simulink model "dqn_C_PQ_HVsMC"  (R2024a)
settings: Solver=FixedStepDiscrete  StartTime=0.0  StopTime=10  FixedStep=Ts_Power  RelTol=1e-3
PreLoadFcn:
  | % HVDCMMCInterconnectionParam
StartFcn:
  | tic
StopFcn:
  | toc
values from neighbouring files (symbols this model uses):
  C_PM = 1.758e-3    (= 0.001758)    [dqnMMCsingle.m]
  Fnom = 50    [dqnMMCsingle.m]
  HRM = 1    [dqnMMCsingle.m]
  Ki_Ireg = 6    [dqnMMCsingle.m]
  Ki_Qreg = 1.0    (= 1)    [dqnMMCsingle.m]
  Kp_Ireg = 0.6    [dqnMMCsingle.m]
  Kp_Qreg = 0.5/3    (= 0.166666666667)    [dqnMMCsingle.m]
  Larm = Larm_pu*(Zb_ac/(2*pi*Fnom))    [dqnMMCsingle.m]
  Larm_pu = 0.15    [dqnMMCsingle.m]
  Lff = Larm_pu/2    (= 0.075)    [dqnMMCsingle.m]
  Limits_Ireg = [ 2.0  -2.0]    [dqnMMCsingle.m]
  Limits_Qreg = [ 0.25, -0.25 ]    [dqnMMCsingle.m]
  Limits_VDCreg = [ 2.0  -2.0]    [dqnMMCsingle.m]
  Lxfo = 0.12    [dqnMMCsingle.m]
  N = 1    [dqnMMCsingle.m]
  Nb_PM = 36    [dqnMMCsingle.m]
  Pnom = 1000e6    (= 1000000000)    [dqnMMCsingle.m]
  R_startup = 400    [dqnMMCsingle.m]
  Rarm = Rarm_pu*Zb_ac    [dqnMMCsingle.m]
  Rff = Rarm_pu/2    (= 0.00075)    [dqnMMCsingle.m]
  Rxfo = 0.003    [dqnMMCsingle.m]
  Slope_Qref = 0.5    [dqnMMCsingle.m]
  Slope_Vdc_ref = Vnom_dc/5    (= 128000)    [dqnMMCsingle.m]
  Tfault = 9999    [dqnMMCsingle.m]
  Ts = Ts_Control    (= 4e-05)    [dqnMMCsingle.m]
  Ts_Control = 40e-6    (= 4e-05)    [dqnMMCsingle.m]
  Ts_dqn = 2e-5    (= 2e-05)    [dqnMMCsingle.m]
  Ts_Power = 20e-6    (= 2e-05)    [dqnMMCsingle.m]
  Vnom_dc = 640e3    (= 640000)    [dqnMMCsingle.m]
  Vnom_prim = 400e3    (= 400000)    [dqnMMCsingle.m]
  Vnom_sec = 333e3    (= 333000)    [dqnMMCsingle.m]
  Ws = 2*pi*50    (= 314.159265359)    [dqnMMCsingle.m]
undefined symbols (not defined in the file or in its folder): DiscIntNeverNeededParam, Discrete, DQN_Lib, gcbh, Int_DQNc_Mat, Mult_DQNc_Mat, Pcc, S, sps, sps_rtmsupport, spsMeanValueVariableFrequencyModel, spsPLL3phModel, SY3
libraries: simulink x18, spsControlledVoltageSourceLib x15, spsVoltageMeasurementLib x9, powerlib_extras x6, spsSecondOrderFilterLib x6, spsCurrentMeasurementLib x6, spsIdealSwitchLib x6, spsMeanLib x4, spsdq0toabcLib x4, spsMeanVariableFrequencyLib x4, spsabctodq0Lib x4, spsThreePhaseSeriesRLCBranchLib x4
(part 6 of 6)

== matlab function dqn_C_PQ_HVsMC/DQsym/Mult_DQNc_Mat3 ==
  data: Xdcpnz_c input; Ydcpnz_c input; N parameter; HrmDbl parameter; Zdcpnz_c output
function Zdcpnz_c    = fMultDQNc(Xdcpnz_c, Ydcpnz_c, N, HrmDbl)
    Zdcpnz_c = complex(zeros(3,2*N+1));

    persistent T132;
    persistent T213;
    persistent T231;
    persistent T321;
    persistent T312;
    persistent Sas;
    persistent Ssa;

    if(isempty(T132)) 
        T132 = [1 0 0; 0 0 1; 0 1 0];
        T213 = [0 1 0; 1 0 0; 0 0 1];
        T231 = [0 1 0; 0 0 1; 1 0 0];
        T321 = [0 0 1; 0 1 0; 1 0 0];
        T312 = [0 0 1; 1 0 0; 0 1 0];

        a = -0.5+0.866i;
        a2 = -0.5-0.866i;
        Sas = [1,a,a2;1,a2,a;1,1,1]/3;
        Ssa = eye(3)/(Sas);
    end

%%%%%%%%%%%%%%%%%%%%%%%%%%%%%%

    Zdcpnz_c(:,1) = Sas*(Ssa*Xdcpnz_c(:,1).*Ssa*Ydcpnz_c(:,1));

    sX = size(Xdcpnz_c,2);
    Xdcpnz_c = [Xdcpnz_c zeros(3,N+1-sX)];

    sY = size(Ydcpnz_c,2);
    Ydcpnz_c = [Ydcpnz_c zeros(3,N+1-sY)];

       
    for h = 1 : 2*N
        if(h<=N)

            Zdcpnz_c(3,1) = Zdcpnz_c(3,1) + 0.5*real(Xdcpnz_c(:,h+1)'*Ydcpnz_c(:,h+1));


            Zdcpnz_c(3,2*h+1) = Zdcpnz_c(3,2*h+1) + 0.5*Xdcpnz_c(1,h+1)*Ydcpnz_c(2,h+1)*exp(-1i*pi/2);

            Zdcpnz_c(1:2,1) = Zdcpnz_c(1:2,1) + 0.25*abs(Xdcpnz_c(1,h+1))*abs(Ydcpnz_c(2,h+1))*[1;1].*exp(1i*((-angle(Xdcpnz_c(1,h+1))+angle(Ydcpnz_c(2,h+1)))*[1;-1]));
            Zdcpnz_c(1:2,1) = Zdcpnz_c(1:2,1) + 0.25*abs(Xdcpnz_c(1,h+1))*abs(Ydcpnz_c(3,h+1))*[1;1].*exp(1i*((-angle(Xdcpnz_c(1,h+1))+angle(Ydcpnz_c(3,h+1)))*[-1;1]));


            Zdcpnz_c(3,2*h+1) = Zdcpnz_c(3,2*h+1) + 0.5*Xdcpnz_c(2,h+1)*Ydcpnz_c(1,h+1)*exp(-1i*pi/2);


            Zdcpnz_c(1:2,1) = Zdcpnz_c(1:2,1) + 0.25*abs(Xdcpnz_c(2,h+1))*abs(Ydcpnz_c(1,h+1))*[1;1].*exp(1i*((-angle(Xdcpnz_c(2,h+1))+angle(Ydcpnz_c(1,h+1)))*[-1;1]));
            Zdcpnz_c(1:2,1) = Zdcpnz_c(1:2,1) + 0.25*abs(Xdcpnz_c(2,h+1))*abs(Ydcpnz_c(3,h+1))*[1;1].*exp(1i*((-angle(Xdcpnz_c(2,h+1))+angle(Ydcpnz_c(3,h+1)))*[1;-1]));
            
            Zdcpnz_c(1:2,1) = Zdcpnz_c(1:2,1) + 0.25*abs(Xdcpnz_c(3,h+1))*abs(Ydcpnz_c(1,h+1))*[1;1].*exp(1i*((-angle(Xdcpnz_c(3,h+1))+angle(Ydcpnz_c(1,h+1)))*[1;-1]));
            Zdcpnz_c(1:2,1) = Zdcpnz_c(1:2,1) + 0.25*abs(Xdcpnz_c(3,h+1))*abs(Ydcpnz_c(2,h+1))*[1;1].*exp(1i*((-angle(Xdcpnz_c(3,h+1))+angle(Ydcpnz_c(2,h+1)))*[-1;+1]));

            %%%%%%%%%%%%%%%%% POSITIVE (Ydc*Xp) %%%%%%%%%%%%%%%%%%%
            Zdcpnz_c(:,h+1) = Zdcpnz_c(:,h+1) + T312*Ydcpnz_c(:,1)*Xdcpnz_c(1,h+1); %[0 0 1; 1 0 0; 0 1 0]
            %%%%%%%%%%%%%%%%% POSITIVE (Xdc*Yp) %%%%%%%%%%%%%%%%%%%
            Zdcpnz_c(:,h+1) = Zdcpnz_c(:,h+1) + T312*Xdcpnz_c(:,1)*Ydcpnz_c(1,h+1);
            %%%%%%%%%%%%%%%%% NEGATIVE (Ydc*Xn) %%%%%%%%%%%%%%%%%%%
            Zdcpnz_c(:,h+1) = Zdcpnz_c(:,h+1) + T231*Ydcpnz_c(:,1)*Xdcpnz_c(2,h+1);
            %%%%%%%%%%%%%%%%% NEGATIVE (Xdc*Yn) %%%%%%%%%%%%%%%%%%%
            Zdcpnz_c(:,h+1) = Zdcpnz_c(:,h+1) + T231*Xdcpnz_c(:,1)*Ydcpnz_c(2,h+1);
            %%%%%%%%%%%%%%%%%%%%%%%%%%%%%%%%%%%%%%%%%%%%%%%%%%%%%%
            Zdcpnz_c(:,h+1) = Zdcpnz_c(:,h+1) + Ydcpnz_c(:,1)*Xdcpnz_c(3,h+1);
            %%%%%%%%%%%%%%%%%%%%%%%%%%%%%%%%%%%%%%%%%%%%%%%%%%%%%%
            Zdcpnz_c(:,h+1) = Zdcpnz_c(:,h+1) + Xdcpnz_c(:,1)*Ydcpnz_c(3,h+1);
            
%%%%%%%%%%%%%%%%%%%%%% h<=N ODD %%%%%%%%%%%%%%%%%%%%%%%%%%%%%%%%%%%%%%%%%
            if(mod(h,2)==1) 
                %%%%%%%%%%%%%%%%% D3p (3ph+) %%%%%%%%%%%%%%%%%%%%%%%

                %&%%%%%%%%%%%%%%%%%%%%%%%%%% PP + NN %%%%%%%%%%%%%%%%%%%%%%%%%%%
                for i = 1 : h - 1
                   Zdcpnz_c(1,h+1) = Zdcpnz_c(1,h+1) +    0.5*( real(Xdcpnz_c(2,i+1))*imag(Ydcpnz_c(2,h-i+1)) + imag(Xdcpnz_c(2,i+1))*real(Ydcpnz_c(2,h-i+1)) );
                   Zdcpnz_c(1,h+1) = Zdcpnz_c(1,h+1) + 1i*0.5*( -real(Xdcpnz_c(2,i+1))*real(Ydcpnz_c(2,h-i+1)) + imag(Xdcpnz_c(2,i+1))*imag(Ydcpnz_c(2,h-i+1)) );

                   Zdcpnz_c(2,h+1) = Zdcpnz_c(2,h+1) +    0.5*( real(Xdcpnz_c(1,i+1))*imag(Ydcpnz_c(1,h-i+1)) + imag(Xdcpnz_c(1,i+1))*real(Ydcpnz_c(1,h-i+1)) );
                   Zdcpnz_c(2,h+1) = Zdcpnz_c(2,h+1) + 1i*0.5*( -real(Xdcpnz_c(1,i+1))*real(Ydcpnz_c(1,h-i+1)) + imag(Xdcpnz_c(1,i+1))*imag(Ydcpnz_c(1,h-i+1)) );
                end

                for i = 1 : N - h

                    Zdcpnz_c(3,h+1) = Zdcpnz_c(3,h+1) -    imag(0.5*Xdcpnz_c(1:2,i+1)'*Ydcpnz_c(1:2,i+h+1)) -    imag(0.5*Ydcpnz_c(1:2,i+1)'*Xdcpnz_c(1:2,i+h+1));
                    Zdcpnz_c(3,h+1) = Zdcpnz_c(3,h+1) + 1i*real(0.5*Xdcpnz_c(1:2,i+1)'*Ydcpnz_c(1:2,i+h+1)) + 1i*real(0.5*Ydcpnz_c(1:2,i+1)'*Xdcpnz_c(1:2,i+h+1));

                end
                %&%%%%%%%%%%%%%%%%%%%%%%%%%% PP + NN %%%%%%%%%%%%%%%%%%%%%%%%%%%

                for k = 1 : (N + mod(N+1,2) - h)/2
                    i = 2*k-1;
                    j = i+h;

                    Zdcpnz_c(1,h+1) = Zdcpnz_c(1,h+1) + (0.5*(Xdcpnz_c(:,i+1)'*T132*T213*Ydcpnz_c(:,j+1))*exp(+1i*pi/2)) ...
                                                      + (0.5*(Xdcpnz_c(:,j+1)'*T213*T132*Ydcpnz_c(:,i+1))*exp(-1i*pi/2))';

                    Zdcpnz_c(2,h+1) = Zdcpnz_c(2,h+1) + (0.5*(Xdcpnz_c(:,i+1)'*T132*T321*Ydcpnz_c(:,j+1))*exp(+1i*pi/2)) ...
                                                      + (0.5*(Xdcpnz_c(:,j+1)'*T321*T132*Ydcpnz_c(:,i+1))*exp(-1i*pi/2))';

                    Zdcpnz_c(3,h+1) = Zdcpnz_c(3,h+1) + (0.5*Xdcpnz_c(3,i+1)'*Ydcpnz_c(3,j+1)*exp(1i*pi/2)) ...
                                                      - (0.5*Xdcpnz_c(3,j+1)'*Ydcpnz_c(3,i+1)*exp(1i*pi/2))';
                end

                for k = 1 : (N + mod(N,2) - h - 1)/2
                    i = 2*k;
                    j = i+h;
                    
                    Zdcpnz_c(1,h+1) = Zdcpnz_c(1,h+1) + (0.5*(Xdcpnz_c(:,i+1)'*T132*T213*Ydcpnz_c(:,j+1))*exp(+1i*pi/2)) ...
                                                      + (0.5*(Xdcpnz_c(:,j+1)'*T213*T132*Ydcpnz_c(:,i+1))*exp(-1i*pi/2))';

                    Zdcpnz_c(2,h+1) = Zdcpnz_c(2,h+1) + (0.5*(Xdcpnz_c(:,i+1)'*T132*T321*Ydcpnz_c(:,j+1))*exp(+1i*pi/2)) ...
                                                      + (0.5*(Xdcpnz_c(:,j+1)'*T321*T132*Ydcpnz_c(:,i+1))*exp(-1i*pi/2))';

                    Zdcpnz_c(3,h+1) = Zdcpnz_c(3,h+1) + (0.5*Xdcpnz_c(3,i+1)'*Ydcpnz_c(3,j+1)*exp(1i*pi/2)) ...
                                                      - (0.5*Xdcpnz_c(3,j+1)'*Ydcpnz_c(3,i+1)*exp(1i*pi/2))';
                end

                for k = (h-1)/2:-1:1
                    i = k;
                    j = h-i;  

                    Zdcpnz_c(3,h+1) = Zdcpnz_c(3,h+1) + 0.5*(real(Xdcpnz_c(:,i+1))'*T213*imag(Ydcpnz_c(:,j+1)) + imag(Xdcpnz_c(:,i+1))'*T213*real(Ydcpnz_c(:,j+1)) ...
                                                           + real(Xdcpnz_c(:,j+1))'*T213*imag(Ydcpnz_c(:,i+1)) + imag(Xdcpnz_c(:,j+1))'*T213*real(Ydcpnz_c(:,i+1)));
                                                                                       
                    Zdcpnz_c(3,h+1) = Zdcpnz_c(3,h+1) + 1i*0.5*(-real(Xdcpnz_c(:,i+1))'*T213*real(Ydcpnz_c(:,j+1)) + imag(Xdcpnz_c(:,i+1))'*T213*imag(Ydcpnz_c(:,j+1)) ...
                                                           - real(Xdcpnz_c(:,j+1))'*T213*real(Ydcpnz_c(:,i+1)) + imag(Xdcpnz_c(:,j+1))'*T213*imag(Ydcpnz_c(:,i+1)));

                    Zdcpnz_c(1,h+1) = Zdcpnz_c(1,h+1) + 0.5*(real(Xdcpnz_c([1,3],i+1))'*[0 1; 1 0]*imag(Ydcpnz_c([1,3],j+1)) + imag(Xdcpnz_c([1,3],i+1))'*[0 1; 1 0]*real(Ydcpnz_c([1,3],j+1)) ...
                                                           + real(Xdcpnz_c([1,3],j+1))'*[0 1; 1 0]*imag(Ydcpnz_c([1,3],i+1)) + imag(Xdcpnz_c([1,3],j+1))'*[0 1; 1 0]*real(Ydcpnz_c([1,3],i+1)) );

                    Zdcpnz_c(1,h+1) = Zdcpnz_c(1,h+1) + 1i*0.5*(-real(Xdcpnz_c([1,3],i+1))'*[0 1; 1 0]*real(Ydcpnz_c([1,3],j+1)) + imag(Xdcpnz_c([1,3],i+1))'*[0 1; 1 0]*imag(Ydcpnz_c([1,3],j+1)) ...
                                                              - real(Xdcpnz_c([1,3],j+1))'*[0 1; 1 0]*real(Ydcpnz_c([1,3],i+1)) + imag(Xdcpnz_c([1,3],j+1))'*[0 1; 1 0]*imag(Ydcpnz_c([1,3],i+1)) );

                    Zdcpnz_c(2,h+1) = Zdcpnz_c(2,h+1) + 0.5*(real(Xdcpnz_c([2,3],i+1))'*[0 1; 1 0]*imag(Ydcpnz_c([2,3],j+1)) + imag(Xdcpnz_c([2,3],i+1))'*[0 1; 1 0]*real(Ydcpnz_c([2,3],j+1)) ...
                                                           + real(Xdcpnz_c([2,3],j+1))'*[0 1; 1 0]*imag(Ydcpnz_c([2,3],i+1)) + imag(Xdcpnz_c([2,3],j+1))'*[0 1; 1 0]*real(Ydcpnz_c([2,3],i+1)) );

                    Zdcpnz_c(2,h+1) = Zdcpnz_c(2,h+1) + 1i*0.5*(-real(Xdcpnz_c([2,3],i+1))'*[0 1; 1 0]*real(Ydcpnz_c([2,3],j+1)) + imag(Xdcpnz_c([2,3],i+1))'*[0 1; 1 0]*imag(Ydcpnz_c([2,3],j+1)) ...
                                                              - real(Xdcpnz_c([2,3],j+1))'*[0 1; 1 0]*real(Ydcpnz_c([2,3],i+1)) + imag(Xdcpnz_c([2,3],j+1))'*[0 1; 1 0]*imag(Ydcpnz_c([2,3],i+1)) );

                end
%%%%%%%%%%%%%%%%%%%%%% h<=N EVEN %%%%%%%%%%%%%%%%%%%%%%%%%%%%%%%%%%%%%%%%%           
            else  

                Zdcpnz_c(3,h+1) = Zdcpnz_c(3,h+1) + 0.5*imag(Xdcpnz_c(3,h/2+1)*Ydcpnz_c(3,h/2+1))           -0.5*1i*real(Xdcpnz_c(3,h/2+1)*Ydcpnz_c(3,h/2+1));
                Zdcpnz_c(1,h+1) = Zdcpnz_c(1,h+1) + 0.5*real(Xdcpnz_c(:,h/2+1))'*T321*imag(Ydcpnz_c(:,h/2+1)) + 0.5*imag(Xdcpnz_c(:,h/2+1))'*T321*real(Ydcpnz_c(:,h/2+1));
                Zdcpnz_c(1,h+1) = Zdcpnz_c(1,h+1) - 0.5*1i*real(Xdcpnz_c(:,h/2+1))'*T321*real(Ydcpnz_c(:,h/2+1)) + 0.5*1i*imag(Xdcpnz_c(:,h/2+1))'*T321*imag(Ydcpnz_c(:,h/2+1));
                Zdcpnz_c(2,h+1) = Zdcpnz_c(2,h+1) + 0.5*real(Xdcpnz_c(:,h/2+1))'*T132*imag(Ydcpnz_c(:,h/2+1)) + 0.5*imag(Xdcpnz_c(:,h/2+1))'*T132*real(Ydcpnz_c(:,h/2+1));
                Zdcpnz_c(2,h+1) = Zdcpnz_c(2,h+1) - 0.5*1i*real(Xdcpnz_c(:,h/2+1))'*T132*real(Ydcpnz_c(:,h/2+1)) + 0.5*1i*imag(Xdcpnz_c(:,h/2+1))'*T132*imag(Ydcpnz_c(:,h/2+1));
                
                for k = 1:N-h
                    i = k;
                    j = h+i;

                    Zdcpnz_c(1,h+1) = Zdcpnz_c(1,h+1) + 0.5*( - real(Xdcpnz_c(:,i+1))'*T231*imag(Ydcpnz_c(:,j+1)) + imag(Xdcpnz_c(:,i+1))'*T231*real(Ydcpnz_c(:,j+1)) ...
                                                              + real(Xdcpnz_c(:,j+1))'*T312*imag(Ydcpnz_c(:,i+1)) - imag(Xdcpnz_c(:,j+1))'*T312*real(Ydcpnz_c(:,i+1)));

                    Zdcpnz_c(1,h+1) = Zdcpnz_c(1,h+1) + 0.5*1i*( + real(Xdcpnz_c(:,i+1))'*T231*real(Ydcpnz_c(:,j+1)) + imag(Xdcpnz_c(:,i+1))'*T231*imag(Ydcpnz_c(:,j+1)) ...
                                                                 + real(Xdcpnz_c(:,j+1))'*T312*real(Ydcpnz_c(:,i+1)) + imag(Xdcpnz_c(:,j+1))'*T312*imag(Ydcpnz_c(:,i+1)));

                    Zdcpnz_c(2,h+1) = Zdcpnz_c(2,h+1) + 0.5*( - real(Xdcpnz_c(:,i+1))'*T312*imag(Ydcpnz_c(:,j+1)) + imag(Xdcpnz_c(:,i+1))'*T312*real(Ydcpnz_c(:,j+1)) ...
                                                              + real(Xdcpnz_c(:,j+1))'*T231*imag(Ydcpnz_c(:,i+1)) - imag(Xdcpnz_c(:,j+1))'*T231*real(Ydcpnz_c(:,i+1)));

                    Zdcpnz_c(2,h+1) = Zdcpnz_c(2,h+1) + 1i*0.5*( + real(Xdcpnz_c(:,i+1))'*T312*real(Ydcpnz_c(:,j+1)) + imag(Xdcpnz_c(:,i+1))'*T312*imag(Ydcpnz_c(:,j+1)) ...
                                                              + real(Xdcpnz_c(:,j+1))'*T231*real(Ydcpnz_c(:,i+1)) + imag(Xdcpnz_c(:,j+1))'*T231*imag(Ydcpnz_c(:,i+1)));

                    Zdcpnz_c(3,h+1) = Zdcpnz_c(3,h+1) + 0.5*(-real(Xdcpnz_c(:,i+1))'*imag(Ydcpnz_c(:,j+1))+imag(Xdcpnz_c(:,i+1))'*real(Ydcpnz_c(:,j+1)) ...
                                                             +real(Xdcpnz_c(:,j+1))'*imag(Ydcpnz_c(:,i+1))-imag(Xdcpnz_c(:,j+1))'*real(Ydcpnz_c(:,i+1)));

                    Zdcpnz_c(3,h+1) = Zdcpnz_c(3,h+1) + 0.5*1i*(+real(Xdcpnz_c(:,i+1))'*real(Ydcpnz_c(:,j+1))+imag(Xdcpnz_c(:,i+1))'*imag(Ydcpnz_c(:,j+1)) ...
                                                             +real(Xdcpnz_c(:,j+1))'*real(Ydcpnz_c(:,i+1))+imag(Xdcpnz_c(:,j+1))'*imag(Ydcpnz_c(:,i+1)));

                end

                for k = h/2-1:-1:1
                    i = k;
                    j = h-i;   

                    Zdcpnz_c(3,h+1) = Zdcpnz_c(3,h+1) +    0.5*(+real(Xdcpnz_c(:,i+1))'*T213*imag(Ydcpnz_c(:,j+1)) + real(Xdcpnz_c(:,j+1))'*T213*imag(Ydcpnz_c(:,i+1)) + imag(Xdcpnz_c(:,i+1))'*T213*real(Ydcpnz_c(:,j+1)) + imag(Xdcpnz_c(:,j+1))'*T213*real(Ydcpnz_c(:,i+1)));

                    Zdcpnz_c(3,h+1) = Zdcpnz_c(3,h+1) + 1i*0.5*(-real(Xdcpnz_c(:,i+1))'*T213*real(Ydcpnz_c(:,j+1)) - real(Xdcpnz_c(:,j+1))'*T213*real(Ydcpnz_c(:,i+1)) + imag(Xdcpnz_c(:,i+1))'*T213*imag(Ydcpnz_c(:,j+1)) + imag(Xdcpnz_c(:,j+1))'*T213*imag(Ydcpnz_c(:,i+1)));

                    Zdcpnz_c(1,h+1) = Zdcpnz_c(1,h+1) + 0.5*( + real(Xdcpnz_c(:,i+1))'*T321*imag(Ydcpnz_c(:,j+1)) + imag(Xdcpnz_c(:,i+1))'*T321*real(Ydcpnz_c(:,j+1)) ...
                                                              + real(Xdcpnz_c(:,j+1))'*T321*imag(Ydcpnz_c(:,i+1)) + imag(Xdcpnz_c(:,j+1))'*T321*real(Ydcpnz_c(:,i+1)));


                    Zdcpnz_c(1,h+1) = Zdcpnz_c(1,h+1) + 0.5*1i*( - real(Xdcpnz_c(:,i+1))'*T321*real(Ydcpnz_c(:,j+1)) + imag(Xdcpnz_c(:,i+1))'*T321*imag(Ydcpnz_c(:,j+1)) ...
                                                                 - real(Xdcpnz_c(:,j+1))'*T321*real(Ydcpnz_c(:,i+1)) + imag(Xdcpnz_c(:,j+1))'*T321*imag(Ydcpnz_c(:,i+1)));
                    
                    Zdcpnz_c(2,h+1) = Zdcpnz_c(2,h+1) + 0.5*( + real(Xdcpnz_c(:,i+1))'*T132*imag(Ydcpnz_c(:,j+1)) + imag(Xdcpnz_c(:,i+1))'*T132*real(Ydcpnz_c(:,j+1)) ...
                                                              + real(Xdcpnz_c(:,j+1))'*T132*imag(Ydcpnz_c(:,i+1)) + imag(Xdcpnz_c(:,j+1))'*T132*real(Ydcpnz_c(:,i+1)));

                    Zdcpnz_c(2,h+1) = Zdcpnz_c(2,h+1) + 1i*0.5*( - real(Xdcpnz_c(:,i+1))'*T132*real(Ydcpnz_c(:,j+1)) + imag(Xdcpnz_c(:,i+1))'*T132*imag(Ydcpnz_c(:,j+1)) ...
                                                                 - real(Xdcpnz_c(:,j+1))'*T132*real(Ydcpnz_c(:,i+1)) + imag(Xdcpnz_c(:,j+1))'*T132*imag(Ydcpnz_c(:,i+1)));

                end
            end
%%%%%%%%%%%%%%%%%%%%%%%%%%%% h>N  %%%%%%%%%%%%%%%%%%%%%%%%%%%%%%%%%%%%%%%%% 
        else %h>N
            if(HrmDbl)
            
                %%%%%%%%%%%%%%%%%%%%%%%%%%% PP + NN %%%%%%%%%%%%%%%%%%%%%%%%%%%
                for i = h-N : N
                    Zdcpnz_c(1,h+1) = Zdcpnz_c(1,h+1) +    0.5*( real(Xdcpnz_c(2,i+1))*imag(Ydcpnz_c(2,h-i+1)) + imag(Xdcpnz_c(2,i+1))*real(Ydcpnz_c(2,h-i+1)) );
                    Zdcpnz_c(1,h+1) = Zdcpnz_c(1,h+1) + 1i*0.5*( -real(Xdcpnz_c(2,i+1))*real(Ydcpnz_c(2,h-i+1)) + imag(Xdcpnz_c(2,i+1))*imag(Ydcpnz_c(2,h-i+1)) );

                    Zdcpnz_c(2,h+1) = Zdcpnz_c(2,h+1) +    0.5*( real(Xdcpnz_c(1,i+1))*imag(Ydcpnz_c(1,h-i+1)) + imag(Xdcpnz_c(1,i+1))*real(Ydcpnz_c(1,h-i+1)) );
                    Zdcpnz_c(2,h+1) = Zdcpnz_c(2,h+1) + 1i*0.5*( -real(Xdcpnz_c(1,i+1))*real(Ydcpnz_c(1,h-i+1)) + imag(Xdcpnz_c(1,i+1))*imag(Ydcpnz_c(1,h-i+1)) );
                end
                %%%%%%%%%%%%%%%%%%%%%%%%%%% PP + NN %%%%%%%%%%%%%%%%%%%%%%%%%%%

                if(mod(h,2)==1) %%%%%%%%%%% h>N ODD %%%%%%%%%%%%%%%%%%%

                    for k = (h-1)/2:-1:h-N
                        i = k;  %%%
                        j = h-i;

                        Zdcpnz_c(1,h+1) = Zdcpnz_c(1,h+1) + 0.5*( + real(Xdcpnz_c([1,3],i+1))'*imag(Ydcpnz_c([3,1],j+1)) + imag(Xdcpnz_c([1,3],i+1))'*real(Ydcpnz_c([3,1],j+1)) ...
                                                                  + real(Xdcpnz_c([1,3],j+1))'*imag(Ydcpnz_c([3,1],i+1)) + imag(Xdcpnz_c([1,3],j+1))'*real(Ydcpnz_c([3,1],i+1)));

                        Zdcpnz_c(1,h+1) = Zdcpnz_c(1,h+1) + 1i*0.5*( - real(Xdcpnz_c([1,3],i+1))'*real(Ydcpnz_c([3,1],j+1)) + imag(Xdcpnz_c([1,3],i+1))'*imag(Ydcpnz_c([3,1],j+1)) ...
                                                                     - real(Xdcpnz_c([1,3],j+1))'*real(Ydcpnz_c([3,1],i+1)) + imag(Xdcpnz_c([1,3],j+1))'*imag(Ydcpnz_c([3,1],i+1)));

                        Zdcpnz_c(2,h+1) = Zdcpnz_c(2,h+1) + 0.5*( + real(Xdcpnz_c([2,3],i+1))'*imag(Ydcpnz_c([3,2],j+1)) + imag(Xdcpnz_c([2,3],i+1))'*real(Ydcpnz_c([3,2],j+1)) ...
                                                                  + real(Xdcpnz_c([2,3],j+1))'*imag(Ydcpnz_c([3,2],i+1)) + imag(Xdcpnz_c([2,3],j+1))'*real(Ydcpnz_c([3,2],i+1)));

                        Zdcpnz_c(2,h+1) = Zdcpnz_c(2,h+1) + 1i*0.5*( - real(Xdcpnz_c([2,3],i+1))'*real(Ydcpnz_c([3,2],j+1)) + imag(Xdcpnz_c([2,3],i+1))'*imag(Ydcpnz_c([3,2],j+1)) ...
                                                                     - real(Xdcpnz_c([2,3],j+1))'*real(Ydcpnz_c([3,2],i+1)) + imag(Xdcpnz_c([2,3],j+1))'*imag(Ydcpnz_c([3,2],i+1)));

                        Zdcpnz_c(3,h+1) = Zdcpnz_c(3,h+1) +    0.5*(+real(Xdcpnz_c(:,i+1))'*T213*imag(Ydcpnz_c(:,j+1)) + real(Xdcpnz_c(:,j+1))'*T213*imag(Ydcpnz_c(:,i+1)) + imag(Xdcpnz_c(:,i+1))'*T213*real(Ydcpnz_c(:,j+1)) + imag(Xdcpnz_c(:,j+1))'*T213*real(Ydcpnz_c(:,i+1)));
                        Zdcpnz_c(3,h+1) = Zdcpnz_c(3,h+1) + 1i*0.5*(-real(Xdcpnz_c(:,i+1))'*T213*real(Ydcpnz_c(:,j+1)) - real(Xdcpnz_c(:,j+1))'*T213*real(Ydcpnz_c(:,i+1)) + imag(Xdcpnz_c(:,i+1))'*T213*imag(Ydcpnz_c(:,j+1)) + imag(Xdcpnz_c(:,j+1))'*T213*imag(Ydcpnz_c(:,i+1)));

                    end

                else %%%%%%%%%%% h>N EVEN %%%%%%%%%%%%%%%%%%%

                    Zdcpnz_c(1,h+1) = 0.5*real(Xdcpnz_c(:,h/2+1))'*T321*imag(Ydcpnz_c(:,h/2+1)) + 0.5*imag(Xdcpnz_c(:,h/2+1))'*T321*real(Ydcpnz_c(:,h/2+1)) - 0.5*1i*real(Xdcpnz_c(:,h/2+1))'*T321*real(Ydcpnz_c(:,h/2+1)) + 0.5*1i*imag(Xdcpnz_c(:,h/2+1))'*T321*imag(Ydcpnz_c(:,h/2+1));
                    Zdcpnz_c(2,h+1) = 0.5*real(Xdcpnz_c(:,h/2+1))'*T132*imag(Ydcpnz_c(:,h/2+1)) + 0.5*imag(Xdcpnz_c(:,h/2+1))'*T132*real(Ydcpnz_c(:,h/2+1))- 0.5*1i*real(Xdcpnz_c(:,h/2+1))'*T132*real(Ydcpnz_c(:,h/2+1)) + 0.5*1i*imag(Xdcpnz_c(:,h/2+1))'*T132*imag(Ydcpnz_c(:,h/2+1));
                    Zdcpnz_c(3,h+1) = Zdcpnz_c(3,h+1) + 0.5*imag(Xdcpnz_c(3,h/2+1)*Ydcpnz_c(3,h/2+1)) - 1i*0.5*real(Xdcpnz_c(3,h/2+1)*Ydcpnz_c(3,h/2+1));


                    for i = (h+2)/2:N
                        j = h-i;

                        Zdcpnz_c(1,h+1) = Zdcpnz_c(1,h+1) + 0.5*( + real(Xdcpnz_c(:,i+1))'*T321*imag(Ydcpnz_c(:,j+1)) + imag(Xdcpnz_c(:,i+1))'*T321*real(Ydcpnz_c(:,j+1)) ...
                                                                  + real(Xdcpnz_c(:,j+1))'*T321*imag(Ydcpnz_c(:,i+1)) + imag(Xdcpnz_c(:,j+1))'*T321*real(Ydcpnz_c(:,i+1)));
    
                        Zdcpnz_c(1,h+1) = Zdcpnz_c(1,h+1) + 0.5*1i*( - real(Xdcpnz_c(:,i+1))'*T321*real(Ydcpnz_c(:,j+1)) + imag(Xdcpnz_c(:,i+1))'*T321*imag(Ydcpnz_c(:,j+1)) ...
                                                                     - real(Xdcpnz_c(:,j+1))'*T321*real(Ydcpnz_c(:,i+1)) + imag(Xdcpnz_c(:,j+1))'*T321*imag(Ydcpnz_c(:,i+1)));

                        Zdcpnz_c(2,h+1) = Zdcpnz_c(2,h+1) + 0.5*( + real(Xdcpnz_c(:,i+1))'*T132*imag(Ydcpnz_c(:,j+1)) + imag(Xdcpnz_c(:,i+1))'*T132*real(Ydcpnz_c(:,j+1)) ...
                                                                  + real(Xdcpnz_c(:,j+1))'*T132*imag(Ydcpnz_c(:,i+1)) + imag(Xdcpnz_c(:,j+1))'*T132*real(Ydcpnz_c(:,i+1)));
    
                        Zdcpnz_c(2,h+1) = Zdcpnz_c(2,h+1) + 0.5*1i*( - real(Xdcpnz_c(:,i+1))'*T132*real(Ydcpnz_c(:,j+1)) + imag(Xdcpnz_c(:,i+1))'*T132*imag(Ydcpnz_c(:,j+1)) ...
                                                                     - real(Xdcpnz_c(:,j+1))'*T132*real(Ydcpnz_c(:,i+1)) + imag(Xdcpnz_c(:,j+1))'*T132*imag(Ydcpnz_c(:,i+1)));

                        Zdcpnz_c(3,h+1) = Zdcpnz_c(3,h+1) +    0.5*(+real(Xdcpnz_c(:,i+1))'*T213*imag(Ydcpnz_c(:,j+1)) + real(Xdcpnz_c(:,j+1))'*T213*imag(Ydcpnz_c(:,i+1)) + imag(Xdcpnz_c(:,i+1))'*T213*real(Ydcpnz_c(:,j+1)) + imag(Xdcpnz_c(:,j+1))'*T213*real(Ydcpnz_c(:,i+1)));
                        Zdcpnz_c(3,h+1) = Zdcpnz_c(3,h+1) + 1i*0.5*(-real(Xdcpnz_c(:,i+1))'*T213*real(Ydcpnz_c(:,j+1)) - real(Xdcpnz_c(:,j+1))'*T213*real(Ydcpnz_c(:,i+1)) + imag(Xdcpnz_c(:,i+1))'*T213*imag(Ydcpnz_c(:,j+1)) + imag(Xdcpnz_c(:,j+1))'*T213*imag(Ydcpnz_c(:,i+1)));

                    end
                end
            end
        end  
    end
    

end

== matlab function dqn_C_PQ_HVsMC/DQsym/Mult_DQNc_Mat4 ==
  data: Xdcpnz_c input; Ydcpnz_c input; N parameter; HrmDbl parameter; Zdcpnz_c output
function Zdcpnz_c    = fMultDQNc(Xdcpnz_c, Ydcpnz_c, N, HrmDbl)
    Zdcpnz_c = complex(zeros(3,2*N+1));

    persistent T132;
    persistent T213;
    persistent T231;
    persistent T321;
    persistent T312;
    persistent Sas;
    persistent Ssa;

    if(isempty(T132)) 
        T132 = [1 0 0; 0 0 1; 0 1 0];
        T213 = [0 1 0; 1 0 0; 0 0 1];
        T231 = [0 1 0; 0 0 1; 1 0 0];
        T321 = [0 0 1; 0 1 0; 1 0 0];
        T312 = [0 0 1; 1 0 0; 0 1 0];

        a = -0.5+0.866i;
        a2 = -0.5-0.866i;
        Sas = [1,a,a2;1,a2,a;1,1,1]/3;
        Ssa = eye(3)/(Sas);
    end

%%%%%%%%%%%%%%%%%%%%%%%%%%%%%%

    Zdcpnz_c(:,1) = Sas*(Ssa*Xdcpnz_c(:,1).*Ssa*Ydcpnz_c(:,1));

    sX = size(Xdcpnz_c,2);
    Xdcpnz_c = [Xdcpnz_c zeros(3,N+1-sX)];

    sY = size(Ydcpnz_c,2);
    Ydcpnz_c = [Ydcpnz_c zeros(3,N+1-sY)];

       
    for h = 1 : 2*N
        if(h<=N)

            Zdcpnz_c(3,1) = Zdcpnz_c(3,1) + 0.5*real(Xdcpnz_c(:,h+1)'*Ydcpnz_c(:,h+1));


            Zdcpnz_c(3,2*h+1) = Zdcpnz_c(3,2*h+1) + 0.5*Xdcpnz_c(1,h+1)*Ydcpnz_c(2,h+1)*exp(-1i*pi/2);

            Zdcpnz_c(1:2,1) = Zdcpnz_c(1:2,1) + 0.25*abs(Xdcpnz_c(1,h+1))*abs(Ydcpnz_c(2,h+1))*[1;1].*exp(1i*((-angle(Xdcpnz_c(1,h+1))+angle(Ydcpnz_c(2,h+1)))*[1;-1]));
            Zdcpnz_c(1:2,1) = Zdcpnz_c(1:2,1) + 0.25*abs(Xdcpnz_c(1,h+1))*abs(Ydcpnz_c(3,h+1))*[1;1].*exp(1i*((-angle(Xdcpnz_c(1,h+1))+angle(Ydcpnz_c(3,h+1)))*[-1;1]));


            Zdcpnz_c(3,2*h+1) = Zdcpnz_c(3,2*h+1) + 0.5*Xdcpnz_c(2,h+1)*Ydcpnz_c(1,h+1)*exp(-1i*pi/2);


            Zdcpnz_c(1:2,1) = Zdcpnz_c(1:2,1) + 0.25*abs(Xdcpnz_c(2,h+1))*abs(Ydcpnz_c(1,h+1))*[1;1].*exp(1i*((-angle(Xdcpnz_c(2,h+1))+angle(Ydcpnz_c(1,h+1)))*[-1;1]));
            Zdcpnz_c(1:2,1) = Zdcpnz_c(1:2,1) + 0.25*abs(Xdcpnz_c(2,h+1))*abs(Ydcpnz_c(3,h+1))*[1;1].*exp(1i*((-angle(Xdcpnz_c(2,h+1))+angle(Ydcpnz_c(3,h+1)))*[1;-1]));
            
            Zdcpnz_c(1:2,1) = Zdcpnz_c(1:2,1) + 0.25*abs(Xdcpnz_c(3,h+1))*abs(Ydcpnz_c(1,h+1))*[1;1].*exp(1i*((-angle(Xdcpnz_c(3,h+1))+angle(Ydcpnz_c(1,h+1)))*[1;-1]));
            Zdcpnz_c(1:2,1) = Zdcpnz_c(1:2,1) + 0.25*abs(Xdcpnz_c(3,h+1))*abs(Ydcpnz_c(2,h+1))*[1;1].*exp(1i*((-angle(Xdcpnz_c(3,h+1))+angle(Ydcpnz_c(2,h+1)))*[-1;+1]));

            %%%%%%%%%%%%%%%%% POSITIVE (Ydc*Xp) %%%%%%%%%%%%%%%%%%%
            Zdcpnz_c(:,h+1) = Zdcpnz_c(:,h+1) + T312*Ydcpnz_c(:,1)*Xdcpnz_c(1,h+1); %[0 0 1; 1 0 0; 0 1 0]
            %%%%%%%%%%%%%%%%% POSITIVE (Xdc*Yp) %%%%%%%%%%%%%%%%%%%
            Zdcpnz_c(:,h+1) = Zdcpnz_c(:,h+1) + T312*Xdcpnz_c(:,1)*Ydcpnz_c(1,h+1);
            %%%%%%%%%%%%%%%%% NEGATIVE (Ydc*Xn) %%%%%%%%%%%%%%%%%%%
            Zdcpnz_c(:,h+1) = Zdcpnz_c(:,h+1) + T231*Ydcpnz_c(:,1)*Xdcpnz_c(2,h+1);
            %%%%%%%%%%%%%%%%% NEGATIVE (Xdc*Yn) %%%%%%%%%%%%%%%%%%%
            Zdcpnz_c(:,h+1) = Zdcpnz_c(:,h+1) + T231*Xdcpnz_c(:,1)*Ydcpnz_c(2,h+1);
            %%%%%%%%%%%%%%%%%%%%%%%%%%%%%%%%%%%%%%%%%%%%%%%%%%%%%%
            Zdcpnz_c(:,h+1) = Zdcpnz_c(:,h+1) + Ydcpnz_c(:,1)*Xdcpnz_c(3,h+1);
            %%%%%%%%%%%%%%%%%%%%%%%%%%%%%%%%%%%%%%%%%%%%%%%%%%%%%%
            Zdcpnz_c(:,h+1) = Zdcpnz_c(:,h+1) + Xdcpnz_c(:,1)*Ydcpnz_c(3,h+1);
            
%%%%%%%%%%%%%%%%%%%%%% h<=N ODD %%%%%%%%%%%%%%%%%%%%%%%%%%%%%%%%%%%%%%%%%
            if(mod(h,2)==1) 
                %%%%%%%%%%%%%%%%% D3p (3ph+) %%%%%%%%%%%%%%%%%%%%%%%

                %&%%%%%%%%%%%%%%%%%%%%%%%%%% PP + NN %%%%%%%%%%%%%%%%%%%%%%%%%%%
                for i = 1 : h - 1
                   Zdcpnz_c(1,h+1) = Zdcpnz_c(1,h+1) +    0.5*( real(Xdcpnz_c(2,i+1))*imag(Ydcpnz_c(2,h-i+1)) + imag(Xdcpnz_c(2,i+1))*real(Ydcpnz_c(2,h-i+1)) );
                   Zdcpnz_c(1,h+1) = Zdcpnz_c(1,h+1) + 1i*0.5*( -real(Xdcpnz_c(2,i+1))*real(Ydcpnz_c(2,h-i+1)) + imag(Xdcpnz_c(2,i+1))*imag(Ydcpnz_c(2,h-i+1)) );

                   Zdcpnz_c(2,h+1) = Zdcpnz_c(2,h+1) +    0.5*( real(Xdcpnz_c(1,i+1))*imag(Ydcpnz_c(1,h-i+1)) + imag(Xdcpnz_c(1,i+1))*real(Ydcpnz_c(1,h-i+1)) );
                   Zdcpnz_c(2,h+1) = Zdcpnz_c(2,h+1) + 1i*0.5*( -real(Xdcpnz_c(1,i+1))*real(Ydcpnz_c(1,h-i+1)) + imag(Xdcpnz_c(1,i+1))*imag(Ydcpnz_c(1,h-i+1)) );
                end

                for i = 1 : N - h

                    Zdcpnz_c(3,h+1) = Zdcpnz_c(3,h+1) -    imag(0.5*Xdcpnz_c(1:2,i+1)'*Ydcpnz_c(1:2,i+h+1)) -    imag(0.5*Ydcpnz_c(1:2,i+1)'*Xdcpnz_c(1:2,i+h+1));
                    Zdcpnz_c(3,h+1) = Zdcpnz_c(3,h+1) + 1i*real(0.5*Xdcpnz_c(1:2,i+1)'*Ydcpnz_c(1:2,i+h+1)) + 1i*real(0.5*Ydcpnz_c(1:2,i+1)'*Xdcpnz_c(1:2,i+h+1));

                end
                %&%%%%%%%%%%%%%%%%%%%%%%%%%% PP + NN %%%%%%%%%%%%%%%%%%%%%%%%%%%

                for k = 1 : (N + mod(N+1,2) - h)/2
                    i = 2*k-1;
                    j = i+h;

                    Zdcpnz_c(1,h+1) = Zdcpnz_c(1,h+1) + (0.5*(Xdcpnz_c(:,i+1)'*T132*T213*Ydcpnz_c(:,j+1))*exp(+1i*pi/2)) ...
                                                      + (0.5*(Xdcpnz_c(:,j+1)'*T213*T132*Ydcpnz_c(:,i+1))*exp(-1i*pi/2))';

                    Zdcpnz_c(2,h+1) = Zdcpnz_c(2,h+1) + (0.5*(Xdcpnz_c(:,i+1)'*T132*T321*Ydcpnz_c(:,j+1))*exp(+1i*pi/2)) ...
                                                      + (0.5*(Xdcpnz_c(:,j+1)'*T321*T132*Ydcpnz_c(:,i+1))*exp(-1i*pi/2))';

                    Zdcpnz_c(3,h+1) = Zdcpnz_c(3,h+1) + (0.5*Xdcpnz_c(3,i+1)'*Ydcpnz_c(3,j+1)*exp(1i*pi/2)) ...
                                                      - (0.5*Xdcpnz_c(3,j+1)'*Ydcpnz_c(3,i+1)*exp(1i*pi/2))';
                end

                for k = 1 : (N + mod(N,2) - h - 1)/2
                    i = 2*k;
                    j = i+h;
                    
                    Zdcpnz_c(1,h+1) = Zdcpnz_c(1,h+1) + (0.5*(Xdcpnz_c(:,i+1)'*T132*T213*Ydcpnz_c(:,j+1))*exp(+1i*pi/2)) ...
                                                      + (0.5*(Xdcpnz_c(:,j+1)'*T213*T132*Ydcpnz_c(:,i+1))*exp(-1i*pi/2))';

                    Zdcpnz_c(2,h+1) = Zdcpnz_c(2,h+1) + (0.5*(Xdcpnz_c(:,i+1)'*T132*T321*Ydcpnz_c(:,j+1))*exp(+1i*pi/2)) ...
                                                      + (0.5*(Xdcpnz_c(:,j+1)'*T321*T132*Ydcpnz_c(:,i+1))*exp(-1i*pi/2))';

                    Zdcpnz_c(3,h+1) = Zdcpnz_c(3,h+1) + (0.5*Xdcpnz_c(3,i+1)'*Ydcpnz_c(3,j+1)*exp(1i*pi/2)) ...
                                                      - (0.5*Xdcpnz_c(3,j+1)'*Ydcpnz_c(3,i+1)*exp(1i*pi/2))';
                end

                for k = (h-1)/2:-1:1
                    i = k;
                    j = h-i;  

                    Zdcpnz_c(3,h+1) = Zdcpnz_c(3,h+1) + 0.5*(real(Xdcpnz_c(:,i+1))'*T213*imag(Ydcpnz_c(:,j+1)) + imag(Xdcpnz_c(:,i+1))'*T213*real(Ydcpnz_c(:,j+1)) ...
                                                           + real(Xdcpnz_c(:,j+1))'*T213*imag(Ydcpnz_c(:,i+1)) + imag(Xdcpnz_c(:,j+1))'*T213*real(Ydcpnz_c(:,i+1)));
                                                                                       
                    Zdcpnz_c(3,h+1) = Zdcpnz_c(3,h+1) + 1i*0.5*(-real(Xdcpnz_c(:,i+1))'*T213*real(Ydcpnz_c(:,j+1)) + imag(Xdcpnz_c(:,i+1))'*T213*imag(Ydcpnz_c(:,j+1)) ...
                                                           - real(Xdcpnz_c(:,j+1))'*T213*real(Ydcpnz_c(:,i+1)) + imag(Xdcpnz_c(:,j+1))'*T213*imag(Ydcpnz_c(:,i+1)));

                    Zdcpnz_c(1,h+1) = Zdcpnz_c(1,h+1) + 0.5*(real(Xdcpnz_c([1,3],i+1))'*[0 1; 1 0]*imag(Ydcpnz_c([1,3],j+1)) + imag(Xdcpnz_c([1,3],i+1))'*[0 1; 1 0]*real(Ydcpnz_c([1,3],j+1)) ...
                                                           + real(Xdcpnz_c([1,3],j+1))'*[0 1; 1 0]*imag(Ydcpnz_c([1,3],i+1)) + imag(Xdcpnz_c([1,3],j+1))'*[0 1; 1 0]*real(Ydcpnz_c([1,3],i+1)) );

                    Zdcpnz_c(1,h+1) = Zdcpnz_c(1,h+1) + 1i*0.5*(-real(Xdcpnz_c([1,3],i+1))'*[0 1; 1 0]*real(Ydcpnz_c([1,3],j+1)) + imag(Xdcpnz_c([1,3],i+1))'*[0 1; 1 0]*imag(Ydcpnz_c([1,3],j+1)) ...
                                                              - real(Xdcpnz_c([1,3],j+1))'*[0 1; 1 0]*real(Ydcpnz_c([1,3],i+1)) + imag(Xdcpnz_c([1,3],j+1))'*[0 1; 1 0]*imag(Ydcpnz_c([1,3],i+1)) );

                    Zdcpnz_c(2,h+1) = Zdcpnz_c(2,h+1) + 0.5*(real(Xdcpnz_c([2,3],i+1))'*[0 1; 1 0]*imag(Ydcpnz_c([2,3],j+1)) + imag(Xdcpnz_c([2,3],i+1))'*[0 1; 1 0]*real(Ydcpnz_c([2,3],j+1)) ...
                                                           + real(Xdcpnz_c([2,3],j+1))'*[0 1; 1 0]*imag(Ydcpnz_c([2,3],i+1)) + imag(Xdcpnz_c([2,3],j+1))'*[0 1; 1 0]*real(Ydcpnz_c([2,3],i+1)) );

                    Zdcpnz_c(2,h+1) = Zdcpnz_c(2,h+1) + 1i*0.5*(-real(Xdcpnz_c([2,3],i+1))'*[0 1; 1 0]*real(Ydcpnz_c([2,3],j+1)) + imag(Xdcpnz_c([2,3],i+1))'*[0 1; 1 0]*imag(Ydcpnz_c([2,3],j+1)) ...
                                                              - real(Xdcpnz_c([2,3],j+1))'*[0 1; 1 0]*real(Ydcpnz_c([2,3],i+1)) + imag(Xdcpnz_c([2,3],j+1))'*[0 1; 1 0]*imag(Ydcpnz_c([2,3],i+1)) );

                end
%%%%%%%%%%%%%%%%%%%%%% h<=N EVEN %%%%%%%%%%%%%%%%%%%%%%%%%%%%%%%%%%%%%%%%%           
            else  

                Zdcpnz_c(3,h+1) = Zdcpnz_c(3,h+1) + 0.5*imag(Xdcpnz_c(3,h/2+1)*Ydcpnz_c(3,h/2+1))           -0.5*1i*real(Xdcpnz_c(3,h/2+1)*Ydcpnz_c(3,h/2+1));
                Zdcpnz_c(1,h+1) = Zdcpnz_c(1,h+1) + 0.5*real(Xdcpnz_c(:,h/2+1))'*T321*imag(Ydcpnz_c(:,h/2+1)) + 0.5*imag(Xdcpnz_c(:,h/2+1))'*T321*real(Ydcpnz_c(:,h/2+1));
                Zdcpnz_c(1,h+1) = Zdcpnz_c(1,h+1) - 0.5*1i*real(Xdcpnz_c(:,h/2+1))'*T321*real(Ydcpnz_c(:,h/2+1)) + 0.5*1i*imag(Xdcpnz_c(:,h/2+1))'*T321*imag(Ydcpnz_c(:,h/2+1));
                Zdcpnz_c(2,h+1) = Zdcpnz_c(2,h+1) + 0.5*real(Xdcpnz_c(:,h/2+1))'*T132*imag(Ydcpnz_c(:,h/2+1)) + 0.5*imag(Xdcpnz_c(:,h/2+1))'*T132*real(Ydcpnz_c(:,h/2+1));
                Zdcpnz_c(2,h+1) = Zdcpnz_c(2,h+1) - 0.5*1i*real(Xdcpnz_c(:,h/2+1))'*T132*real(Ydcpnz_c(:,h/2+1)) + 0.5*1i*imag(Xdcpnz_c(:,h/2+1))'*T132*imag(Ydcpnz_c(:,h/2+1));
                
                for k = 1:N-h
                    i = k;
                    j = h+i;

                    Zdcpnz_c(1,h+1) = Zdcpnz_c(1,h+1) + 0.5*( - real(Xdcpnz_c(:,i+1))'*T231*imag(Ydcpnz_c(:,j+1)) + imag(Xdcpnz_c(:,i+1))'*T231*real(Ydcpnz_c(:,j+1)) ...
                                                              + real(Xdcpnz_c(:,j+1))'*T312*imag(Ydcpnz_c(:,i+1)) - imag(Xdcpnz_c(:,j+1))'*T312*real(Ydcpnz_c(:,i+1)));

                    Zdcpnz_c(1,h+1) = Zdcpnz_c(1,h+1) + 0.5*1i*( + real(Xdcpnz_c(:,i+1))'*T231*real(Ydcpnz_c(:,j+1)) + imag(Xdcpnz_c(:,i+1))'*T231*imag(Ydcpnz_c(:,j+1)) ...
                                                                 + real(Xdcpnz_c(:,j+1))'*T312*real(Ydcpnz_c(:,i+1)) + imag(Xdcpnz_c(:,j+1))'*T312*imag(Ydcpnz_c(:,i+1)));

                    Zdcpnz_c(2,h+1) = Zdcpnz_c(2,h+1) + 0.5*( - real(Xdcpnz_c(:,i+1))'*T312*imag(Ydcpnz_c(:,j+1)) + imag(Xdcpnz_c(:,i+1))'*T312*real(Ydcpnz_c(:,j+1)) ...
                                                              + real(Xdcpnz_c(:,j+1))'*T231*imag(Ydcpnz_c(:,i+1)) - imag(Xdcpnz_c(:,j+1))'*T231*real(Ydcpnz_c(:,i+1)));

                    Zdcpnz_c(2,h+1) = Zdcpnz_c(2,h+1) + 1i*0.5*( + real(Xdcpnz_c(:,i+1))'*T312*real(Ydcpnz_c(:,j+1)) + imag(Xdcpnz_c(:,i+1))'*T312*imag(Ydcpnz_c(:,j+1)) ...
                                                              + real(Xdcpnz_c(:,j+1))'*T231*real(Ydcpnz_c(:,i+1)) + imag(Xdcpnz_c(:,j+1))'*T231*imag(Ydcpnz_c(:,i+1)));

                    Zdcpnz_c(3,h+1) = Zdcpnz_c(3,h+1) + 0.5*(-real(Xdcpnz_c(:,i+1))'*imag(Ydcpnz_c(:,j+1))+imag(Xdcpnz_c(:,i+1))'*real(Ydcpnz_c(:,j+1)) ...
                                                             +real(Xdcpnz_c(:,j+1))'*imag(Ydcpnz_c(:,i+1))-imag(Xdcpnz_c(:,j+1))'*real(Ydcpnz_c(:,i+1)));

                    Zdcpnz_c(3,h+1) = Zdcpnz_c(3,h+1) + 0.5*1i*(+real(Xdcpnz_c(:,i+1))'*real(Ydcpnz_c(:,j+1))+imag(Xdcpnz_c(:,i+1))'*imag(Ydcpnz_c(:,j+1)) ...
                                                             +real(Xdcpnz_c(:,j+1))'*real(Ydcpnz_c(:,i+1))+imag(Xdcpnz_c(:,j+1))'*imag(Ydcpnz_c(:,i+1)));

                end

                for k = h/2-1:-1:1
                    i = k;
                    j = h-i;   

                    Zdcpnz_c(3,h+1) = Zdcpnz_c(3,h+1) +    0.5*(+real(Xdcpnz_c(:,i+1))'*T213*imag(Ydcpnz_c(:,j+1)) + real(Xdcpnz_c(:,j+1))'*T213*imag(Ydcpnz_c(:,i+1)) + imag(Xdcpnz_c(:,i+1))'*T213*real(Ydcpnz_c(:,j+1)) + imag(Xdcpnz_c(:,j+1))'*T213*real(Ydcpnz_c(:,i+1)));

                    Zdcpnz_c(3,h+1) = Zdcpnz_c(3,h+1) + 1i*0.5*(-real(Xdcpnz_c(:,i+1))'*T213*real(Ydcpnz_c(:,j+1)) - real(Xdcpnz_c(:,j+1))'*T213*real(Ydcpnz_c(:,i+1)) + imag(Xdcpnz_c(:,i+1))'*T213*imag(Ydcpnz_c(:,j+1)) + imag(Xdcpnz_c(:,j+1))'*T213*imag(Ydcpnz_c(:,i+1)));

                    Zdcpnz_c(1,h+1) = Zdcpnz_c(1,h+1) + 0.5*( + real(Xdcpnz_c(:,i+1))'*T321*imag(Ydcpnz_c(:,j+1)) + imag(Xdcpnz_c(:,i+1))'*T321*real(Ydcpnz_c(:,j+1)) ...
                                                              + real(Xdcpnz_c(:,j+1))'*T321*imag(Ydcpnz_c(:,i+1)) + imag(Xdcpnz_c(:,j+1))'*T321*real(Ydcpnz_c(:,i+1)));


                    Zdcpnz_c(1,h+1) = Zdcpnz_c(1,h+1) + 0.5*1i*( - real(Xdcpnz_c(:,i+1))'*T321*real(Ydcpnz_c(:,j+1)) + imag(Xdcpnz_c(:,i+1))'*T321*imag(Ydcpnz_c(:,j+1)) ...
                                                                 - real(Xdcpnz_c(:,j+1))'*T321*real(Ydcpnz_c(:,i+1)) + imag(Xdcpnz_c(:,j+1))'*T321*imag(Ydcpnz_c(:,i+1)));
                    
                    Zdcpnz_c(2,h+1) = Zdcpnz_c(2,h+1) + 0.5*( + real(Xdcpnz_c(:,i+1))'*T132*imag(Ydcpnz_c(:,j+1)) + imag(Xdcpnz_c(:,i+1))'*T132*real(Ydcpnz_c(:,j+1)) ...
                                                              + real(Xdcpnz_c(:,j+1))'*T132*imag(Ydcpnz_c(:,i+1)) + imag(Xdcpnz_c(:,j+1))'*T132*real(Ydcpnz_c(:,i+1)));

                    Zdcpnz_c(2,h+1) = Zdcpnz_c(2,h+1) + 1i*0.5*( - real(Xdcpnz_c(:,i+1))'*T132*real(Ydcpnz_c(:,j+1)) + imag(Xdcpnz_c(:,i+1))'*T132*imag(Ydcpnz_c(:,j+1)) ...
                                                                 - real(Xdcpnz_c(:,j+1))'*T132*real(Ydcpnz_c(:,i+1)) + imag(Xdcpnz_c(:,j+1))'*T132*imag(Ydcpnz_c(:,i+1)));

                end
            end
%%%%%%%%%%%%%%%%%%%%%%%%%%%% h>N  %%%%%%%%%%%%%%%%%%%%%%%%%%%%%%%%%%%%%%%%% 
        else %h>N
            if(HrmDbl)
            
                %%%%%%%%%%%%%%%%%%%%%%%%%%% PP + NN %%%%%%%%%%%%%%%%%%%%%%%%%%%
                for i = h-N : N
                    Zdcpnz_c(1,h+1) = Zdcpnz_c(1,h+1) +    0.5*( real(Xdcpnz_c(2,i+1))*imag(Ydcpnz_c(2,h-i+1)) + imag(Xdcpnz_c(2,i+1))*real(Ydcpnz_c(2,h-i+1)) );
                    Zdcpnz_c(1,h+1) = Zdcpnz_c(1,h+1) + 1i*0.5*( -real(Xdcpnz_c(2,i+1))*real(Ydcpnz_c(2,h-i+1)) + imag(Xdcpnz_c(2,i+1))*imag(Ydcpnz_c(2,h-i+1)) );

                    Zdcpnz_c(2,h+1) = Zdcpnz_c(2,h+1) +    0.5*( real(Xdcpnz_c(1,i+1))*imag(Ydcpnz_c(1,h-i+1)) + imag(Xdcpnz_c(1,i+1))*real(Ydcpnz_c(1,h-i+1)) );
                    Zdcpnz_c(2,h+1) = Zdcpnz_c(2,h+1) + 1i*0.5*( -real(Xdcpnz_c(1,i+1))*real(Ydcpnz_c(1,h-i+1)) + imag(Xdcpnz_c(1,i+1))*imag(Ydcpnz_c(1,h-i+1)) );
                end
                %%%%%%%%%%%%%%%%%%%%%%%%%%% PP + NN %%%%%%%%%%%%%%%%%%%%%%%%%%%

                if(mod(h,2)==1) %%%%%%%%%%% h>N ODD %%%%%%%%%%%%%%%%%%%

                    for k = (h-1)/2:-1:h-N
                        i = k;  %%%
                        j = h-i;

                        Zdcpnz_c(1,h+1) = Zdcpnz_c(1,h+1) + 0.5*( + real(Xdcpnz_c([1,3],i+1))'*imag(Ydcpnz_c([3,1],j+1)) + imag(Xdcpnz_c([1,3],i+1))'*real(Ydcpnz_c([3,1],j+1)) ...
                                                                  + real(Xdcpnz_c([1,3],j+1))'*imag(Ydcpnz_c([3,1],i+1)) + imag(Xdcpnz_c([1,3],j+1))'*real(Ydcpnz_c([3,1],i+1)));

                        Zdcpnz_c(1,h+1) = Zdcpnz_c(1,h+1) + 1i*0.5*( - real(Xdcpnz_c([1,3],i+1))'*real(Ydcpnz_c([3,1],j+1)) + imag(Xdcpnz_c([1,3],i+1))'*imag(Ydcpnz_c([3,1],j+1)) ...
                                                                     - real(Xdcpnz_c([1,3],j+1))'*real(Ydcpnz_c([3,1],i+1)) + imag(Xdcpnz_c([1,3],j+1))'*imag(Ydcpnz_c([3,1],i+1)));

                        Zdcpnz_c(2,h+1) = Zdcpnz_c(2,h+1) + 0.5*( + real(Xdcpnz_c([2,3],i+1))'*imag(Ydcpnz_c([3,2],j+1)) + imag(Xdcpnz_c([2,3],i+1))'*real(Ydcpnz_c([3,2],j+1)) ...
                                                                  + real(Xdcpnz_c([2,3],j+1))'*imag(Ydcpnz_c([3,2],i+1)) + imag(Xdcpnz_c([2,3],j+1))'*real(Ydcpnz_c([3,2],i+1)));

                        Zdcpnz_c(2,h+1) = Zdcpnz_c(2,h+1) + 1i*0.5*( - real(Xdcpnz_c([2,3],i+1))'*real(Ydcpnz_c([3,2],j+1)) + imag(Xdcpnz_c([2,3],i+1))'*imag(Ydcpnz_c([3,2],j+1)) ...
                                                                     - real(Xdcpnz_c([2,3],j+1))'*real(Ydcpnz_c([3,2],i+1)) + imag(Xdcpnz_c([2,3],j+1))'*imag(Ydcpnz_c([3,2],i+1)));

                        Zdcpnz_c(3,h+1) = Zdcpnz_c(3,h+1) +    0.5*(+real(Xdcpnz_c(:,i+1))'*T213*imag(Ydcpnz_c(:,j+1)) + real(Xdcpnz_c(:,j+1))'*T213*imag(Ydcpnz_c(:,i+1)) + imag(Xdcpnz_c(:,i+1))'*T213*real(Ydcpnz_c(:,j+1)) + imag(Xdcpnz_c(:,j+1))'*T213*real(Ydcpnz_c(:,i+1)));
                        Zdcpnz_c(3,h+1) = Zdcpnz_c(3,h+1) + 1i*0.5*(-real(Xdcpnz_c(:,i+1))'*T213*real(Ydcpnz_c(:,j+1)) - real(Xdcpnz_c(:,j+1))'*T213*real(Ydcpnz_c(:,i+1)) + imag(Xdcpnz_c(:,i+1))'*T213*imag(Ydcpnz_c(:,j+1)) + imag(Xdcpnz_c(:,j+1))'*T213*imag(Ydcpnz_c(:,i+1)));

                    end

                else %%%%%%%%%%% h>N EVEN %%%%%%%%%%%%%%%%%%%

                    Zdcpnz_c(1,h+1) = 0.5*real(Xdcpnz_c(:,h/2+1))'*T321*imag(Ydcpnz_c(:,h/2+1)) + 0.5*imag(Xdcpnz_c(:,h/2+1))'*T321*real(Ydcpnz_c(:,h/2+1)) - 0.5*1i*real(Xdcpnz_c(:,h/2+1))'*T321*real(Ydcpnz_c(:,h/2+1)) + 0.5*1i*imag(Xdcpnz_c(:,h/2+1))'*T321*imag(Ydcpnz_c(:,h/2+1));
                    Zdcpnz_c(2,h+1) = 0.5*real(Xdcpnz_c(:,h/2+1))'*T132*imag(Ydcpnz_c(:,h/2+1)) + 0.5*imag(Xdcpnz_c(:,h/2+1))'*T132*real(Ydcpnz_c(:,h/2+1))- 0.5*1i*real(Xdcpnz_c(:,h/2+1))'*T132*real(Ydcpnz_c(:,h/2+1)) + 0.5*1i*imag(Xdcpnz_c(:,h/2+1))'*T132*imag(Ydcpnz_c(:,h/2+1));
                    Zdcpnz_c(3,h+1) = Zdcpnz_c(3,h+1) + 0.5*imag(Xdcpnz_c(3,h/2+1)*Ydcpnz_c(3,h/2+1)) - 1i*0.5*real(Xdcpnz_c(3,h/2+1)*Ydcpnz_c(3,h/2+1));


                    for i = (h+2)/2:N
                        j = h-i;

                        Zdcpnz_c(1,h+1) = Zdcpnz_c(1,h+1) + 0.5*( + real(Xdcpnz_c(:,i+1))'*T321*imag(Ydcpnz_c(:,j+1)) + imag(Xdcpnz_c(:,i+1))'*T321*real(Ydcpnz_c(:,j+1)) ...
                                                                  + real(Xdcpnz_c(:,j+1))'*T321*imag(Ydcpnz_c(:,i+1)) + imag(Xdcpnz_c(:,j+1))'*T321*real(Ydcpnz_c(:,i+1)));
    
                        Zdcpnz_c(1,h+1) = Zdcpnz_c(1,h+1) + 0.5*1i*( - real(Xdcpnz_c(:,i+1))'*T321*real(Ydcpnz_c(:,j+1)) + imag(Xdcpnz_c(:,i+1))'*T321*imag(Ydcpnz_c(:,j+1)) ...
                                                                     - real(Xdcpnz_c(:,j+1))'*T321*real(Ydcpnz_c(:,i+1)) + imag(Xdcpnz_c(:,j+1))'*T321*imag(Ydcpnz_c(:,i+1)));

                        Zdcpnz_c(2,h+1) = Zdcpnz_c(2,h+1) + 0.5*( + real(Xdcpnz_c(:,i+1))'*T132*imag(Ydcpnz_c(:,j+1)) + imag(Xdcpnz_c(:,i+1))'*T132*real(Ydcpnz_c(:,j+1)) ...
                                                                  + real(Xdcpnz_c(:,j+1))'*T132*imag(Ydcpnz_c(:,i+1)) + imag(Xdcpnz_c(:,j+1))'*T132*real(Ydcpnz_c(:,i+1)));
    
                        Zdcpnz_c(2,h+1) = Zdcpnz_c(2,h+1) + 0.5*1i*( - real(Xdcpnz_c(:,i+1))'*T132*real(Ydcpnz_c(:,j+1)) + imag(Xdcpnz_c(:,i+1))'*T132*imag(Ydcpnz_c(:,j+1)) ...
                                                                     - real(Xdcpnz_c(:,j+1))'*T132*real(Ydcpnz_c(:,i+1)) + imag(Xdcpnz_c(:,j+1))'*T132*imag(Ydcpnz_c(:,i+1)));

                        Zdcpnz_c(3,h+1) = Zdcpnz_c(3,h+1) +    0.5*(+real(Xdcpnz_c(:,i+1))'*T213*imag(Ydcpnz_c(:,j+1)) + real(Xdcpnz_c(:,j+1))'*T213*imag(Ydcpnz_c(:,i+1)) + imag(Xdcpnz_c(:,i+1))'*T213*real(Ydcpnz_c(:,j+1)) + imag(Xdcpnz_c(:,j+1))'*T213*real(Ydcpnz_c(:,i+1)));
                        Zdcpnz_c(3,h+1) = Zdcpnz_c(3,h+1) + 1i*0.5*(-real(Xdcpnz_c(:,i+1))'*T213*real(Ydcpnz_c(:,j+1)) - real(Xdcpnz_c(:,j+1))'*T213*real(Ydcpnz_c(:,i+1)) + imag(Xdcpnz_c(:,i+1))'*T213*imag(Ydcpnz_c(:,j+1)) + imag(Xdcpnz_c(:,j+1))'*T213*imag(Ydcpnz_c(:,i+1)));

                    end
                end
            end
        end  
    end
    

end

== matlab function dqn_C_PQ_HVsMC/Control _DQn/PLL, Measurements and Transformation1/MATLAB Function ==
  data: DQ input; wt input; d output; q output
function [d, q] = correct_dq(DQ, wt)
    % Function to calculate phase angle from dq components, correct it, and adjust dq components
    % Inputs:
    %   d, q - Direct and Quadrature axis components
    %   theta_offset - Correction angle (in radians)
    % Outputs:
    %   theta_dq - Original computed dq phase
    %   theta_corrected - Corrected dq phase
    %   d_corrected, q_corrected - Corrected dq components
    d= DQ(1,1);
    q= DQ(2,1);
    % Compute the instantaneous phase angle
    % theta_dq = atan2(q,d);  % atan2 ensures correct quadrant selection
    
    % Apply the phase correction
    % theta_corrected = theta_dq - wt;
    
    % Compute corrected dq components using inverse rotation
    d =   DQ(1,1) * cos(wt) + DQ(2,1) * sin(wt);
    q = - DQ(1,1)  * sin(wt) + DQ(2,1) * cos(wt);
end

== matlab function dqn_C_PQ_HVsMC/Control _DQn/PLL, Measurements and Transformation1/MATLAB Function1 ==
  data: DQ input; wt input; d output; q output
function [d, q] = correct_dq(DQ, wt)
    % Function to calculate phase angle from dq components, correct it, and adjust dq components
    % Inputs:
    %   d, q - Direct and Quadrature axis components
    %   theta_offset - Correction angle (in radians)
    % Outputs:
    %   theta_dq - Original computed dq phase
    %   theta_corrected - Corrected dq phase
    %   d_corrected, q_corrected - Corrected dq components
    d= DQ(1,1);
    q= DQ(2,1);
    % Compute the instantaneous phase angle
    % theta_dq = atan2(q,d);  % atan2 ensures correct quadrant selection
    
    % Apply the phase correction
    % theta_corrected = theta_dq - wt;
    
    % Compute corrected dq components using inverse rotation
    d =   DQ(1,1) * cos(wt) + DQ(2,1) * sin(wt);
    q = - DQ(1,1)  * sin(wt) + DQ(2,1) * cos(wt);
end

== matlab function dqn_C_PQ_HVsMC/Control _DQn/PLL, Measurements and Transformation1/MATLAB Function2 ==
  data: dq input; theta_offset input; d_corrected output; q_corrected output
function [d_corrected, q_corrected] = correct_dq(dq, theta_offset)
    % Function to calculate phase angle from dq components, correct it, and adjust dq components
    % Inputs:
    %   d, q - Direct and Quadrature axis components
    %   theta_offset - Correction angle (in radians)
    % Outputs:
    %   theta_dq - Original computed dq phase
    %   theta_corrected - Corrected dq phase
    %   d_corrected, q_corrected - Corrected dq components
    d= dq(1,1);
    q= dq(2,1);
    % Compute the instantaneous phase angle
    theta_dq = atan2(q,d);  % atan2 ensures correct quadrant selection
    
    % Apply the phase correction
    theta_corrected = theta_dq - theta_offset;
    
    % Compute corrected dq components using inverse rotation
    d_corrected = d * cos(theta_offset) + q * sin(theta_offset);
    q_corrected = -d * sin(theta_offset) + q * cos(theta_offset);
end

== matlab function dqn_C_PQ_HVsMC/Control _DQn/PLL, Measurements and Transformation1/PLL (3ph)2/Model/MATLAB Function ==
  data: DQ input; wt input; d output; q output
function [d, q] = correct_dq(DQ, wt)
    % Function to calculate phase angle from dq components, correct it, and adjust dq components
    % Inputs:
    %   d, q - Direct and Quadrature axis components
    %   theta_offset - Correction angle (in radians)
    % Outputs:
    %   theta_dq - Original computed dq phase
    %   theta_corrected - Corrected dq phase
    %   d_corrected, q_corrected - Corrected dq components
    d= DQ(1,1);
    q= DQ(2,1);
    % Compute the instantaneous phase angle
    % theta_dq = atan2(q,d);  % atan2 ensures correct quadrant selection
    
    % Apply the phase correction
    % theta_corrected = theta_dq - wt;
    
    % Compute corrected dq components using inverse rotation
    d =   DQ(1,1) * cos(wt) + DQ(2,1) * sin(wt);
    q = - DQ(1,1)  * sin(wt) + DQ(2,1) * cos(wt);
end

== matlab function dqn_C_PQ_HVsMC/DQn->ABC ==
  settings: updateMethod=DISCRETE
  data: Xdcpnz_c input; tho input; Xabc output; N parameter
%function abc = Mult(Z0,Zdp,Zqp,Zdn,Zqn,Zdz,Zqz,th, N)
function Xabc = dqn2abc(Xdcpnz_c,tho,N)

    persistent Sas;
    persistent Ssa;

    if(isempty(Sas)) 
        a = -0.5+0.866i;
        a2 = -0.5-0.866i;
        Sas = [1,a,a2;1,a2,a;1,1,1]/3;
        Ssa = eye(3)/(Sas);
    end

    Xabc = zeros(3,1);

    for i = 1 : N+1
    
    
        if(i>1)
            h = i-1;
    
            th = h*tho;
        
            mag_p = abs(Xdcpnz_c(1,i));
            ang_p = angle(Xdcpnz_c(1,i));
            mag_n = abs(Xdcpnz_c(2,i));
            ang_n = angle(Xdcpnz_c(2,i));
            mag_z = abs(Xdcpnz_c(3,i));
            ang_z = angle(Xdcpnz_c(3,i));
            
            abc3p = mag_p*[sin(th+ang_p) ; sin(th+ang_p-2*pi/3) ; sin(th+ang_p+2*pi/3) ];
            abc3n = mag_n*[sin(th+ang_n) ; sin(th+ang_n+2*pi/3) ; sin(th+ang_n-2*pi/3) ];
            abc3z = mag_z*[sin(th+ang_z) ; sin(th+ang_z)        ; sin(th+ang_z)  ];
        
            Xabc = Xabc + abc3p+abc3n+abc3z;
        else
            Xabc = Xabc + real(Ssa*(Xdcpnz_c(:,1)));
        
        end
    
        
    end

end

== matlab function dqn_C_PQ_HVsMC/DQsym/Subsystem/DQn->ABC10 ==
  settings: updateMethod=DISCRETE
  data: Xdcpnz_c input; tho input; Xabc output; N parameter
%function abc = Mult(Z0,Zdp,Zqp,Zdn,Zqn,Zdz,Zqz,th, N)
function Xabc = dqn2abc(Xdcpnz_c,tho,N)

    persistent Sas;
    persistent Ssa;

    if(isempty(Sas)) 
        a = -0.5+0.866i;
        a2 = -0.5-0.866i;
        Sas = [1,a,a2;1,a2,a;1,1,1]/3;
        Ssa = eye(3)/(Sas);
    end

    Xabc = zeros(3,1);

    for i = 1 : N+1
    
    
        if(i>1)
            h = i-1;
    
            th = h*tho;
        
            mag_p = abs(Xdcpnz_c(1,i));
            ang_p = angle(Xdcpnz_c(1,i));
            mag_n = abs(Xdcpnz_c(2,i));
            ang_n = angle(Xdcpnz_c(2,i));
            mag_z = abs(Xdcpnz_c(3,i));
            ang_z = angle(Xdcpnz_c(3,i));
            
            abc3p = mag_p*[sin(th+ang_p) ; sin(th+ang_p-2*pi/3) ; sin(th+ang_p+2*pi/3) ];
            abc3n = mag_n*[sin(th+ang_n) ; sin(th+ang_n+2*pi/3) ; sin(th+ang_n-2*pi/3) ];
            abc3z = mag_z*[sin(th+ang_z) ; sin(th+ang_z)        ; sin(th+ang_z)  ];
        
            Xabc = Xabc + abc3p+abc3n+abc3z;
        else
            Xabc = Xabc + real(Ssa*(Xdcpnz_c(:,1)));
        
        end
    
        
    end

end
